simulink model "lab05"  (Simulink 10.3)
settings: Solver=FixedStepAuto  StartTime=0.0  StopTime=2  FixedStep=0.001768  RelTol=1e-3
values from neighbouring files (symbols this model uses):
  k_d = 0.00416035381008    [lab03.mat]    (also in lab04.mat = 0.00114359359927; lab05.mat = 0.00883154670201; lab06.mat = 0.05; lab07.mat = 0.00883154670201)
  k_p = 2    [lab02.mat]    (also in lab03.mat = 0.256097247605; lab04.mat = 0.137612608424; lab05.mat = 0.280842058008; lab06.mat = 0.012)
  k_pfc = 108.810811765    [lab05.mat]    (also in lab06.mat = 171.157754285; lab07.mat)
undefined symbols (not defined in the file or in its folder): D_ax, G_p, N_ax, R, S
settings Model: Creator=kisdev  LastModifiedBy=kisdev
settings SolverCC: AlgebraicLoopSolver=Auto
settings DataIOCC: SaveFormat=Dataset  SignalLoggingSaveFormat=Dataset  ReturnWorkspaceOutputs=on
settings OptimizationCC: ExpressionDepthLimit=128  LifeSpan=auto
settings DebuggingCC: UnderspecifiedInitializationDetection=Simplified  MergeDetectMultiDrivingBlocksExec=error  FcnCallInpInsideContextMsg=error  StateNameClashWarn=none  SFUnexpectedBacktrackingDiag=error  SFNoUnconditionalDefaultTransitionDiag=error  SFExecutionAtInitializationDiag=warning  SFMachineParentedDataDiag=error  ArithmeticOperatorsInVariantConditions=error
settings HardwareCC: ProdBitPerPointer=64  ProdBitPerSizeT=64  ProdBitPerPtrDiffT=64  ProdLargestAtomicFloat=Float  ProdIntDivRoundTo=Zero  ProdEndianess=LittleEndian  ProdWordSize=64  ProdHWDeviceType=Intel->x86-64 (Windows64)
settings ModelReferenceCC: PropagateSignalLabelsOutOfModel=on
settings SFSimCC: SimUseLocalCustomCode=on  CustomCodeUndefinedFunction=FilterOut
settings RTWCC: RTWUseLocalCustomCode=on
settings CodeAppCC: StateflowObjectComments=off
settings GRTTargetCC: TargetLangStandard=C99 (ISO)  CombineOutputUpdateFcns=on  GRTInterface=off
settings ConfigComp: CovMetricSettings=dwe  CovSaveCumulativeToWorkspaceVar=off  CovSaveSingleToWorkspaceVar=off  CovExternalEMLEnable=on

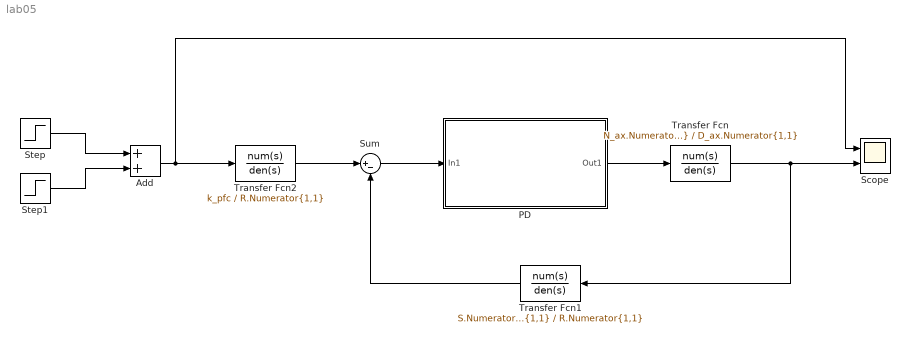
== system lab05 ==
  Add : Sum
  PD : Subsystem
  Scope : Scope  NumInputPorts=2
  Step : Step  Time=0  After=500  SampleTime=0
  Step1 : Step  Time=2.5  After=-1000  SampleTime=0
  Sum : Sum  Inputs=|+-
  Transfer Fcn : TransferFcn  Numerator=N_ax.Numerator{1,1}  Denominator=D_ax.Numerator{1,1}
  Transfer Fcn1 : TransferFcn  Numerator=S.Numerator{1,1}  Denominator=R.Numerator{1,1}
  Transfer Fcn2 : TransferFcn  Numerator=k_pfc  Denominator=R.Numerator{1,1}
  wires:
  Add/1 -> Transfer Fcn2/1, Scope/1
  Step/1 -> Add/1
  Step1/1 -> Add/2
  PD/1(Out1) -> Transfer Fcn/1
  Transfer Fcn/1 -> Transfer Fcn1/1, Scope/2
  Transfer Fcn1/1 -> Sum/2
  Sum/1 -> PD/1(In1)
  Transfer Fcn2/1 -> Sum/1

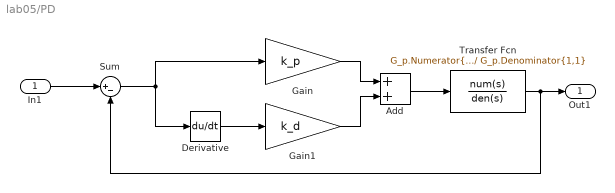
== system lab05/PD ==
  In1 : Inport
  Add : Sum
  Derivative : Derivative
  Gain : Gain  Gain=k_p
  Gain1 : Gain  Gain=k_d
  Sum : Sum  Inputs=|+-
  Transfer Fcn : TransferFcn  Numerator=G_p.Numerator{1,1}  Denominator=G_p.Denominator{1,1}
  Out1 : Outport
  wires:
  Transfer Fcn/1 -> Sum/2, Out1/1
  Gain/1 -> Add/1
  Gain1/1 -> Add/2
  Derivative/1 -> Gain1/1
  In1/1 -> Sum/1
  Sum/1 -> Derivative/1, Gain/1
  Add/1 -> Transfer Fcn/1
